simulink model "DT_vehicle_model"  (R2018a)
settings: Solver=FixedStepDiscrete  StartTime=0.0  StopTime=inf  FixedStep=Tsmall  RelTol=1e-3
PreLoadFcn:
  | DT_data
PostLoadFcn:
  | , if any(exist('dsrtsu_mdlpostloadfcn', 'file') == [2, 3, 6]), try dsrtsu_mdlpostloadfcn('Execute', bdroot); catch fprintf('Error in PostLoadFcn (dsrtsu_mdlpostloadfcn) for model "%s":\n %s\n', bdroot, lasterr); end, end,
InitFcn:
  | DT_data
values from neighbouring files (symbols this model uses):
  Bx_ash_f = 11.7    [DT_data.m]
  Bx_ash_r = 11.1    [DT_data.m]
  Bx_snow_f = 10.2    [DT_data.m]
  Bx_snow_r = 9.71    [DT_data.m]
  By_ash_f = 8.86    [DT_data.m]
  By_ash_r = 9.30    (= 9.3)    [DT_data.m]
  By_snow_f = 19.1    [DT_data.m]
  By_snow_r = 20.0    (= 20)    [DT_data.m]
  Cx_ash_f = 1.69    [DT_data.m]
  Cx_ash_r = 1.69    [DT_data.m]
  Cx_snow_f = 1.96    [DT_data.m]
  Cx_snow_r = 1.96    [DT_data.m]
  Cy_ash_f = 1.19    [DT_data.m]
  Cy_ash_r = 1.19    [DT_data.m]
  Cy_snow_f = 0.550    (= 0.55)    [DT_data.m]
  Cy_snow_r = 0.550    (= 0.55)    [DT_data.m]
  D_phi = 16000    [DT_data.m]
  D_theta = 30960    [DT_data.m]
  delta_r = 0    [DT_data.m]
  epsilon = 0.4    [DT_data.m]
  Ex_ash_f = 0.377    [DT_data.m]
  Ex_ash_r = 0.362    [DT_data.m]
  Ex_snow_f = 0.651    [DT_data.m]
  Ex_snow_r = 0.624    [DT_data.m]
  Ey_ash_f = -1.21    [DT_data.m]
  Ey_ash_r = -1.11    [DT_data.m]
  Ey_snow_f = -2.1    [DT_data.m]
  Ey_snow_r = -1.93    [DT_data.m]
  g = 9.81    [DT_data.m]
  h = 0.5    [DT_data.m]
  Iw = 4    [DT_data.m]
  Ixx = 602.1923    [DT_data.m]
  Iyy = 2.7370e+03    (= 2737)    [DT_data.m]
  Izz = 3070    [DT_data.m]
  K_phi = 178000    [DT_data.m]
  K_theta = 363540    [DT_data.m]
  l_f = 1.2110    (= 1.211)    [DT_data.m]
  l_r = 1.4590    (= 1.459)    [DT_data.m]
  m = 1830    [DT_data.m]
  mu_x_ash_f = 1.20    (= 1.2)    [DT_data.m]
  mu_x_ash_r = 1.20    (= 1.2)    [DT_data.m]
  mu_x_snow_f = 0.407    [DT_data.m]
  mu_x_snow_r = 0.409    [DT_data.m]
  mu_y_ash_f = 0.935    [DT_data.m]
  mu_y_ash_r = 0.961    [DT_data.m]
  mu_y_snow_f = 0.383    [DT_data.m]
  mu_y_snow_r = 0.394    [DT_data.m]
  omega0 = 29.1545    [DT_data.m]
  road = 1    [DT_data.m]
  Rw = 0.3430    (= 0.343)    [DT_data.m]
  Ts = 0.001    [DT_data.m]
  Tsmall = 0.001    [DT_data.m]
  Vx0 = 10    [DT_data.m]
  w = 0.7700    (= 0.77)    [DT_data.m]
libraries: simulink x1
(part 1 of 2)
PreSaveFcn:
  | , if any(exist('dsmpb_private', 'file') == [2, 3, 6]), try, dsmpb_private('dsmpb_mdlclblib', 'PreSave', bdroot); catch, disp(lasterr); end, end,
CloseFcn:
  | , if any(exist('dsmpb_private', 'file') == [2, 3, 6]), try, dsmpb_private('dsmpb_mdlclblib', 'Close', bdroot); catch, disp(lasterr); end, end,
Description:
  | Standard RTI1401 template.
  | Supported MATLAB version:  R2017b.
settings Model: Tag=RTI1401  DSRTSU_INTERNAL_RTI_VER=520  DSRTSU_INTERNAL_RTI_TYPE=rti1006  RTICANMMDATA=struct('GeneralSetupData',struct('modelroot','C:\Users\srivats\Documents\MATLAB\DT_vehicle_model','generalsettings',struct('filesettings',struct('destfolder',struct('Name','RTICANMM_FILES','Check',1),'buildfolder',struct('Name','.','Check',1),'AbsDestfolder',struct('Name','C:\Users\srivats\Documents\MATLAB\DT_vehicle_model\RTICANMM_FILES'),'AbsBuildfolder',struct('Name','C:\Users\srivats\Documents\MATLAB\DT_vehicle_model'))),'options',struct('addpaths',1,'rmpaths',1,'addtrcexclusion',logical(1),'cannavigator',struct('checkmonitoring',0),'show_usrtrc',0,'use_usrtrc',0),'advanced',struct('options',[1 1 1 1 1 1 1 1 1 1 1 1 1 1 1 1 1 1 1 1 1 1 1 1 1 1 1 1 1 1 1 1 1 1 1 1 1 1 1 1 1 1 1 1 1 1 1 1 1 1 1 1 1 1 1 1 1 1 1 1 1 1 1 1 1 1 1 1 1 1 1 1 1 1 1 1 1 1 1 1 1 1 1 1 1 1 1 1 1 1 1 1 1 1 1 1 1 1 1 1]),'MPSetup',{{}},'modelname','DT_vehicle_model','block','DT_vehicle_model'))  DSRTSU_INTERNAL_RTIFLEXRAYCONFIG=110  DSRTSU_INTERNAL_RTIFPGA=110  DSMPB_DATASERVER_ModelPortLibVersion1=8  DSMPB_DATASERVER_DataServerVersion1=6  DSMPB_DATASERVER_DataServerStreamVersion1=3  Creator=merl  LastModifiedBy=srivats
settings OptimizationCC: BlockReduction=off  BooleanDataType=off  ConditionallyExecuteInputs=off  OptimizeBlockIOStorage=off  BufferReuse=off  GlobalBufferReuse=off  ExpressionFolding=off  LocalBlockOutputs=off  OptimizeDataStoreBuffers=off  BusAssignmentInplaceUpdate=off
settings DebuggingCC: MultiTaskRateTransMsg=warning  UnknownTsInhSupMsg=error
settings HardwareCC: ProdBitPerPointer=32  ProdBitPerSizeT=32  ProdBitPerPtrDiffT=32  ProdLargestAtomicInteger=Integer  ProdWordSize=32  ProdHWDeviceType=Custom Processor->Custom  TargetIntDivRoundTo=Zero  TargetEndianess=LittleEndian  TargetHWDeviceType=Custom Processor->Custom
settings SFSimCC: MATLABDynamicMemAlloc=off
settings RTWCC: SystemTargetFile=rti1006.tlc  MakeCommand=make_rti  TemplateMakefile=rti1006.tmf  Description=<inactive> dSPACE DS1006 Hardware Platform
settings CodeAppCC: StateflowObjectComments=on
settings STFCustomTargetCC: ParMdlRefBuildCompliant=on  GRTInterface=off  SystemTargetFile=rti1006.tlc
settings GRTTargetCC: TargetLangStandard=C89/C90 (ANSI)  CompOptLevelCompliant=off  ConcurrentExecutionCompliant=off  CombineOutputUpdateFcns=off  MatFileLogging=off  CPPClassGenCompliant=off  UseToolchainInfoCompliant=off
settings ConfigComp: CovMetricSettings=dswe

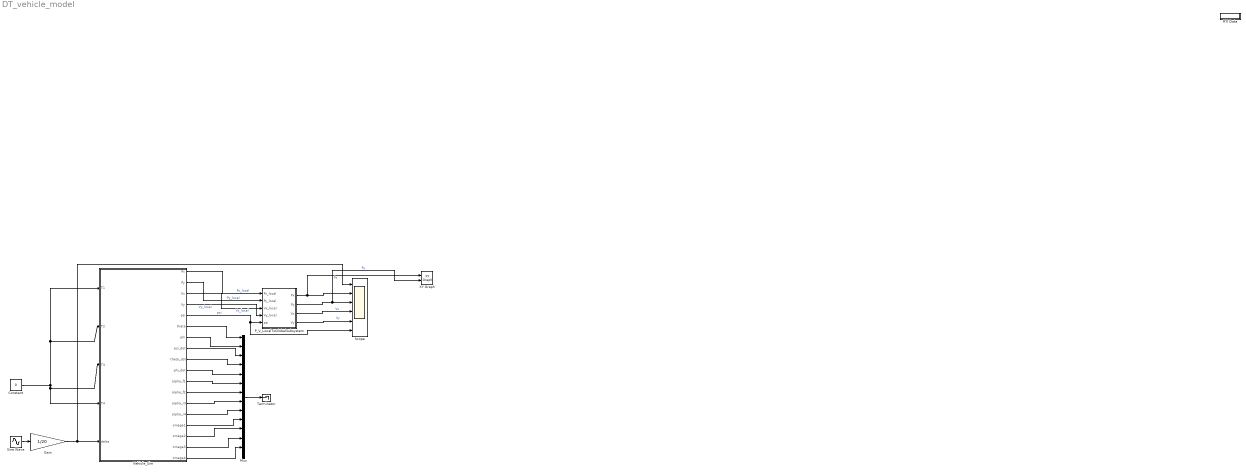
== system DT_vehicle_model ==
  Constant : Constant  Value=0
  Gain : Gain  Gain=1/20
  Mux : Mux  Inputs=14
  P_V_LocalToGlobalSubsystem : Subsystem
  RTI Data : Subsystem  Tag=struct('RTIDataServer',struct('RTIDataServerVs','2','RTIModelDescription','struct(''main'',''DT_vehicle_model'',''sub'','''',''isMp'',0)'))  LoadFcn="if exist('rtidc'), try,  rtidc('DataHostBlockClbLoad', gcbh); catch, disp(['Warning: ''LoadFcn'' for RTI Data block failed: ' lasterr]); end, end,"  mask(RTI_DATA_HOST){}
      mask help:
      | RTI Data Block.
      | This block is used by RTI to store internal model-dependent data.
      | Please keep this block on the root level of the model. Deleting this block will result in data loss.
      |
      | NEVER DELETE OR COPY THIS BLOCK!
      settings: CopyFcn="if exist('rtidc'), try,  rtidc('DataHostBlockClbCopy', gcbh); catch, disp(['Warning: ''CopyFcn'' for RTI Data block failed: ' lasterr]); end, end,"  DeleteFcn="if exist('rtidc'), try,  rtidc('DataHostBlockClbDelete', gcbh); catch, disp(['Warning: ''DeleteFcn'' for RTI Data block failed: ' lasterr]); end, end,"  ModelCloseFcn="if exist('rtidc'), try,  rtidc('DataHostBlockClbModelClose', gcbh); catch, disp(['Warning: ''ModelCloseFcn'' for RTI Data block failed: ' lasterr]); end, end,"  PreSaveFcn="if exist('rtidc'), try,  rtidc('DataHostBlockClbPreSave', gcbh); catch, disp(['Warning: ''PreSaveFcn'' for RTI Data block failed: ' lasterr]); end, end,"  PostSaveFcn="if exist('rtidc'), try,  rtidc('DataHostBlockClbPostSave', gcbh); catch, disp(['Warning: ''PostSaveFcn'' for RTI Data block failed: ' lasterr]); end, end,"  NameChangeFcn="if exist('rtidc'), try,  rtidc('DataHostBlockClbNameChange', gcbh); catch, disp(['Warning: ''NameChangeFcn'' for RTI Data block failed: ' lasterr]); end, end,"
      mask Help:
      | RTI Data Block.
      | This block is used by RTI to store internal model-dependent data.
      | Please keep this block on the root level of the model. Deleting this block will result in data loss.
      | 
      | NEVER DELETE OR COPY THIS BLOCK!
      mask Display:
      | text(0.5, 0.5, 'RTI Data', 'HorizontalAlignment', 'center');
      | plot([1 0]);
  Scope : Scope  NumInputPorts=6
  Sine Wave : Sin  Amplitude=0.5  SampleTime=0
  Terminator : Terminator
  Vehicle_Sim : Subsystem
  XY Graph : simulink/Sinks/XY Graph  xmin=-1000  xmax=1000  ymin=-1000  ymax=1000  st=-1
  wires:
  Vehicle_Sim/6(theta) -> Mux/1
  Vehicle_Sim/7(phi) -> Mux/2
  Vehicle_Sim/8(psi_dot) -> Mux/3
  Vehicle_Sim/9(theta_dot) -> Mux/4
  Vehicle_Sim/10(phi_dot) -> Mux/5
  Vehicle_Sim/11(alpha_f1) -> Mux/6
  Vehicle_Sim/12(alpha_f2) -> Mux/7
  Vehicle_Sim/13(alpha_r3) -> Mux/8
  Vehicle_Sim/14(alpha_r4) -> Mux/9
  Vehicle_Sim/15(omega1) -> Mux/10
  Vehicle_Sim/16(omega2) -> Mux/11
  Vehicle_Sim/17(omega3) -> Mux/12
  Vehicle_Sim/18(omega4) -> Mux/13
  Mux/1 -> Terminator/1
  Sine Wave/1 -> Gain/1
  Vehicle_Sim/1(Px) -> P_V_LocalToGlobalSubsystem/1(Px_local)  "Px_local"
  Vehicle_Sim/2(Py) -> P_V_LocalToGlobalSubsystem/2(Py_local)  "Py_local"
  Vehicle_Sim/3(Vx) -> P_V_LocalToGlobalSubsystem/3(Vx_local)  "Vx_local"
  Vehicle_Sim/4(Vy) -> P_V_LocalToGlobalSubsystem/4(Vy_local)  "Vy_local"
  Vehicle_Sim/5(psi) -> Scope/6, P_V_LocalToGlobalSubsystem/5(psi)  "psi"
  P_V_LocalToGlobalSubsystem/1(Px) -> XY Graph/1, Scope/2  "Px"
  P_V_LocalToGlobalSubsystem/2(Py) -> XY Graph/2, Scope/3  "Py"
  P_V_LocalToGlobalSubsystem/3(Vx) -> Scope/4  "Vx"
  P_V_LocalToGlobalSubsystem/4(Vy) -> Scope/5  "Vy"
  Constant/1 -> Vehicle_Sim/2(T2), Vehicle_Sim/1(T1), Vehicle_Sim/4(T4), Vehicle_Sim/3(T3)
  Gain/1 -> Scope/1, Vehicle_Sim/5("delta ")

== system DT_vehicle_model/P_V_LocalToGlobalSubsystem ==
  Px_local : Inport  OutDataTypeStr=double  SampleTime=Ts
  Py_local : Inport  Port=2  OutDataTypeStr=double  SampleTime=Ts
  Vx_local : Inport  Port=3  OutDataTypeStr=double  SampleTime=Ts
  Vy_local : Inport  Port=4  OutDataTypeStr=double  SampleTime=Ts
  psi : Inport  Port=5  OutDataTypeStr=double  SampleTime=Ts
  Add : Sum  Inputs=+-
  Add1 : Sum
  Add2 : Sum  Inputs=+-
  Add3 : Sum
  Cos : Trigonometry  Operator=cos
  Product{,1..7} (8 alike) : Product
  Sin : Trigonometry
  Px : Outport  OutDataTypeStr=double  SampleTime=Ts
  Py : Outport  Port=2  OutDataTypeStr=double  SampleTime=Ts
  Vx : Outport  Port=3  OutDataTypeStr=double  SampleTime=Ts
  Vy : Outport  Port=4  OutDataTypeStr=double  SampleTime=Ts
  wires:
  Px_local/1 -> Product6/1, Product4/1  "Px_local"
  Py_local/1 -> Product7/1, Product5/1  "Py_local"
  Vx_local/1 -> Product2/1, Product/2  "Vx_local"
  Product5/1 -> Add2/2
  Product4/1 -> Add2/1
  Add2/1 -> Px/1  "Px"
  Product7/1 -> Add3/2
  Vy_local/1 -> Product3/1, Product1/2  "Vy_local"
  psi/1 -> Sin/1, Cos/1  "psi"
  Cos/1 -> Product3/2, Product/1, Product7/2, Product4/2  "cosPsi"
  Add3/1 -> Py/1  "Py"
  Product2/1 -> Add1/1
  Product1/1 -> Add/2
  Add/1 -> Vx/1  "Vx"
  Add1/1 -> Vy/1  "Vy"
  Product6/1 -> Add3/1
  Product3/1 -> Add1/2
  Product/1 -> Add/1
  Sin/1 -> Product2/2, Product1/1, Product6/2, Product5/2  "sinPsi"

== system DT_vehicle_model/RTI Data ==
  RTI Data Store : Subsystem  Tag="struct('private',struct('version',struct('dsVer',uint32(2),'dsVerCreation',uint32(2),'RTI',struct('ver','7.10','type','RTI1006')),'access',struct('type','Model','isPerm',1,'created',['01-Nov-2018 15:30:42'],'modified',['05-Apr-2019 15:16:55'],'location','')),'public',struct('main',struct('data',[]),'sub',struct('name',{{'DT_vehicle_model'}},'data',{{struct('TH',struct('thTaskInfo',struct('taskType',{'TIMER','HWINT','TMRINT','SWINT','GLINT'},'tasksNumOf',{1,0,0,0,0},'srcIds',{{'TIMERA'},{},{},{},{}},'taskNames',{{['Timer Task 1']},{},{},{},{}})),'th_tc',struct('dataType','TASK','taskGroupId','','taskGroupList',{{}},'taskSchedulingPolicy','FCFS','taskType','TIMER','blkh',-1,'srcId','TIMERA','srcSgnName',['Timer A interrupt'],'srcCpuName','','taskName',['Timer Task 1  [0.001] s'],'taskNameDisplayExt','','smplTime',0.001,'smplTimeOffs',0,'hasFixedPriority',0,'priority',1,'hasFixedOvc',0,'ovcType',1,'ovcMax',1),'tc_th',struct('dataType','TASK','taskGroupId','','taskGroupList',{{}},'taskSchedulingPolicy','FCFS','taskType','TIMER','blkh',-1,'srcId','TIMERA','srcSgnName',['Timer A interrupt'],'srcCpuName','','taskName',['Timer Task 1  [0.001] s'],'taskNameDisplayExt','','smplTime',0.001,'smplTimeOffs',0,'hasFixedPriority',0,'priority',1,'hasFixedOvc',0,'ovcType',1,'ovcMax',1))}})))"  mask(RTI_DATA_STORE){}
      mask help:
      | RTI Data Store Block. This block is used by RTI to store internal model dependent data. Deleting this block will result in data loss.
      |
      | NEVER DELETE, COPY, OR MODIFY THIS BLOCK!
      mask Help:
      | RTI Data Store Block. This block is used by RTI to store internal model dependent data. Deleting this block will result in data loss.
      | 
      | NEVER DELETE, COPY, OR MODIFY THIS BLOCK!
      mask Display: text(0.5, 0.5, ' ', 'HorizontalAlignment', 'center');

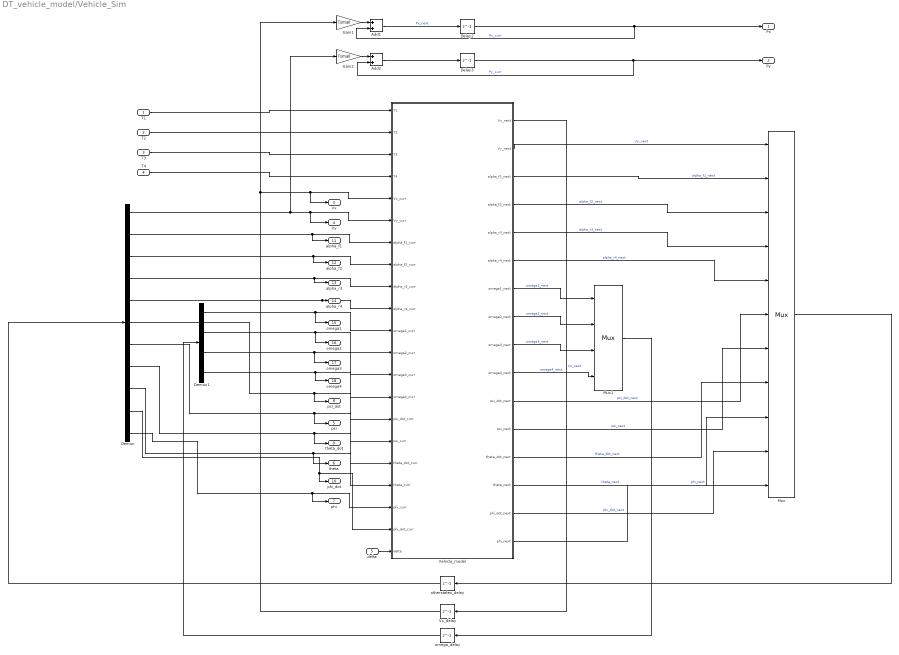
== system DT_vehicle_model/Vehicle_Sim ==
  T1 : Inport  OutDataTypeStr=double  SampleTime=Ts
  T2 : Inport  Port=2  OutDataTypeStr=double  SampleTime=Ts
  T3 : Inport  Port=3  OutDataTypeStr=double  SampleTime=Ts
  T4 : Inport  Port=4  OutDataTypeStr=double  SampleTime=Ts
  "delta " : Inport  Port=5
  Add1 : Sum
  Add2 : Sum
  Delay2 : Delay  DelayLength=1  SampleTime=Tsmall
  Delay3 : Delay  DelayLength=1  SampleTime=Tsmall
  Demux : Demux  Outputs=11
  Demux1 : Demux
  Gain1 : Gain  Gain=Tsmall
  Gain2 : Gain  Gain=Tsmall
  Mux : Mux  Inputs=11
      settings: DisplayOption=signals
  Mux1 : Mux
      settings: DisplayOption=signals
  Vehicle_model : Subsystem
  Vx_delay : Delay  DelayLength=1  InitialCondition=Vx0  SampleTime=Tsmall
  omega_delay : Delay  DelayLength=1  InitialCondition=omega0*ones(4,1)  SampleTime=Tsmall
  otherstates_delay : Delay  DelayLength=1  InitialCondition=zeros(11,1)  SampleTime=Tsmall
  Px : Outport  OutDataTypeStr=double  SampleTime=Tsmall
  Py : Outport  Port=2  OutDataTypeStr=double  SampleTime=Tsmall
  Vx : Outport  Port=3  OutDataTypeStr=double  SampleTime=Tsmall
  Vy : Outport  Port=4  OutDataTypeStr=double  SampleTime=Tsmall
  psi : Outport  Port=5  OutDataTypeStr=double  SampleTime=Tsmall
  theta : Outport  Port=6  OutDataTypeStr=double  SampleTime=Tsmall
  phi : Outport  Port=7  OutDataTypeStr=double  SampleTime=Tsmall
  psi_dot : Outport  Port=8  OutDataTypeStr=double  SampleTime=Tsmall
  theta_dot : Outport  Port=9  OutDataTypeStr=double  SampleTime=Tsmall
  phi_dot : Outport  Port=10  OutDataTypeStr=double  SampleTime=Tsmall
  alpha_f1 : Outport  Port=11  OutDataTypeStr=double  SampleTime=Tsmall
  alpha_f2 : Outport  Port=12  OutDataTypeStr=double  SampleTime=Tsmall
  alpha_r3 : Outport  Port=13  OutDataTypeStr=double  SampleTime=Tsmall
  alpha_r4 : Outport  Port=14  OutDataTypeStr=double  SampleTime=Tsmall
  omega1 : Outport  Port=15  OutDataTypeStr=double  SampleTime=Tsmall
  omega2 : Outport  Port=16  OutDataTypeStr=double  SampleTime=Tsmall
  omega3 : Outport  Port=17  OutDataTypeStr=double  SampleTime=Tsmall
  omega4 : Outport  Port=18  OutDataTypeStr=double  SampleTime=Tsmall
  wires:
  Vehicle_model/14(theta_next) -> Mux/9  "theta_next"
  Vehicle_model/12(psi_next) -> Mux/7  "psi_next"
  Vehicle_model/11(psi_dot_next) -> Mux/6  "psi_dot_next"
  Vehicle_model/15(phi_dot_next) -> Mux/10  "phi_dot_next"
  Mux/1 -> otherstates_delay/1
  Vehicle_model/3(alpha_f1_next) -> Mux/2  "alpha_f1_next"
  Vehicle_model/5(alpha_r3_next) -> Mux/4  "alpha_r3_next"
  Vehicle_model/9(omega3_next) -> Mux1/3  "omega3_next"
  Vehicle_model/8(omega2_next) -> Mux1/2  "omega2_next"
  Vehicle_model/13(theta_dot_next) -> Mux/8  "theta_dot_next"
  Vehicle_model/4(alpha_f2_next) -> Mux/3  "alpha_f2_next"
  Vehicle_model/6(alpha_r4_next) -> Mux/5  "alpha_r4_next"
  Vehicle_model/10(omega4_next) -> Mux1/4  "omega4_next"
  Vehicle_model/1(Vx_next) -> Vx_delay/1  "Vx_next"
  Demux/1 -> Gain2/1, Vy/1, Vehicle_model/6(Vy_curr)
  Vehicle_model/7(omega1_next) -> Mux1/1  "omega1_next"
  Demux1/3 -> omega3/1, Vehicle_model/13(omega3_curr)
  Demux/5 -> Vehicle_model/10(alpha_r4_curr), alpha_r4/1
  Demux/8 -> theta_dot/1, Vehicle_model/17(theta_dot_curr)
  Vehicle_model/16(phi_next) -> Mux/11  "phi_next"
  Vehicle_model/2(Vy_next) -> Mux/1  "Vy_next"
  T1/1 -> Vehicle_model/1(T1)
  Add2/1 -> Delay3/1
  Delay3/1 -> Py/1, Add2/2  "Py_curr"
  Add1/1 -> Delay2/1  "Px_next"
  Delay2/1 -> Px/1, Add1/2  "Px_curr"
  Gain1/1 -> Add1/1
  Gain2/1 -> Add2/1
  T3/1 -> Vehicle_model/3(T3)
  T4/1 -> Vehicle_model/4(T4)
  T2/1 -> Vehicle_model/2(T2)
  otherstates_delay/1 -> Demux/1
  Demux/4 -> Vehicle_model/9(alpha_r3_curr), alpha_r3/1
  Demux/11 -> phi/1, Vehicle_model/19(phi_curr)
  Demux/2 -> Vehicle_model/7(alpha_f1_curr), alpha_f1/1
  Demux/3 -> Vehicle_model/8(alpha_f2_curr), alpha_f2/1
  Demux1/4 -> omega4/1, Vehicle_model/14(omega4_curr)
  Demux/7 -> psi/1, Vehicle_model/16(psi_curr)
  Demux/9 -> theta/1, Vehicle_model/18(theta_curr)
  Demux/10 -> phi_dot/1, Vehicle_model/20(phi_dot_curr)
  Demux/6 -> psi_dot/1, Vehicle_model/15(psi_dot_curr)
  Demux1/2 -> omega2/1, Vehicle_model/12(omega2_curr)
  Vx_delay/1 -> Vx/1, Vehicle_model/5(Vx_curr), Gain1/1
  Demux1/1 -> omega1/1, Vehicle_model/11(omega1_curr)
  Mux1/1 -> omega_delay/1
  omega_delay/1 -> Demux1/1
  "delta "/1 -> Vehicle_model/21(delta)

== system DT_vehicle_model/RTI Data/RTI Data Store ==
  RTI Data Store : Subsystem  mask(RTI_DATA_STORE){}
      mask help:
      | RTI Data Store Block. This block is used by RTI to store internal model dependent data. Deleting this block will result in data loss.
      |
      | NEVER DELETE, COPY, OR MODIFY THIS BLOCK!
      mask Help:
      | RTI Data Store Block. This block is used by RTI to store internal model dependent data. Deleting this block will result in data loss.
      | 
      | NEVER DELETE, COPY, OR MODIFY THIS BLOCK!
      mask Display: text(0.5, 0.5, ' ', 'HorizontalAlignment', 'center');

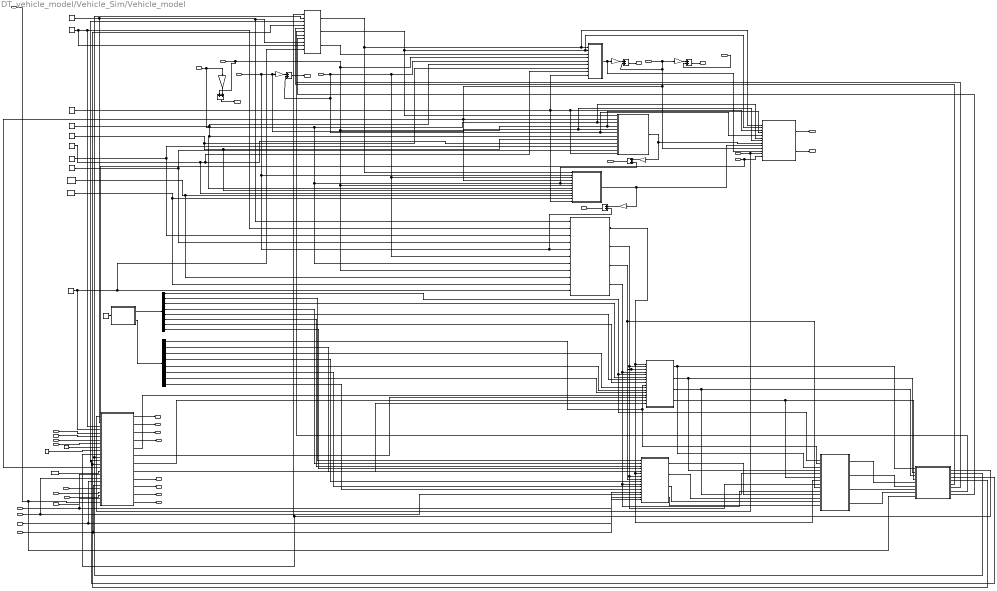
== system DT_vehicle_model/Vehicle_Sim/Vehicle_model ==
  T1 : Inport  OutDataTypeStr=double  SampleTime=Ts
  T2 : Inport  Port=2  OutDataTypeStr=double  SampleTime=Ts
  T3 : Inport  Port=3  OutDataTypeStr=double  SampleTime=Ts
  T4 : Inport  Port=4  OutDataTypeStr=double  SampleTime=Ts
  Vx_curr : Inport  Port=5  OutDataTypeStr=double  SampleTime=Tsmall
  Vy_curr : Inport  Port=6  OutDataTypeStr=double  SampleTime=Tsmall
  alpha_f1_curr : Inport  Port=7  OutDataTypeStr=double  SampleTime=Tsmall
  alpha_f2_curr : Inport  Port=8  OutDataTypeStr=double  SampleTime=Tsmall
  alpha_r3_curr : Inport  Port=9  OutDataTypeStr=double  SampleTime=Tsmall
  alpha_r4_curr : Inport  Port=10  OutDataTypeStr=double  SampleTime=Tsmall
  omega1_curr : Inport  Port=11  OutDataTypeStr=double  SampleTime=Tsmall
  omega2_curr : Inport  Port=12  OutDataTypeStr=double  SampleTime=Tsmall
  omega3_curr : Inport  Port=13  OutDataTypeStr=double  SampleTime=Tsmall
  omega4_curr : Inport  Port=14  OutDataTypeStr=double  SampleTime=Tsmall
  psi_dot_curr : Inport  Port=15  OutDataTypeStr=double  SampleTime=Tsmall
  psi_curr : Inport  Port=16  OutDataTypeStr=double  SampleTime=Tsmall
  theta_dot_curr : Inport  Port=17  OutDataTypeStr=double  SampleTime=Tsmall
  theta_curr : Inport  Port=18  OutDataTypeStr=double  SampleTime=Tsmall
  phi_curr : Inport  Port=19  OutDataTypeStr=double  SampleTime=Tsmall
  phi_dot_curr : Inport  Port=20  OutDataTypeStr=double  SampleTime=Tsmall
  delta : Inport  Port=21  OutDataTypeStr=double  SampleTime=Tsmall
  Add{,1..5} (6 alike) : Sum
  D_phi : Constant  Value=D_phi
  D_theta : Constant  Value=D_theta
  Demux1 : Demux  Outputs=8
  Demux2 : Demux  Outputs=8
  F_M_subsystem : Subsystem
  Fx0_Subsystem : Subsystem
  Fy0_Subsystem : Subsystem
  Fy0_to_Fy_subsystem : Subsystem
  Fz_Subsystem : Subsystem
  Gain{,1..5} (6 alike) : Gain  Gain=Tsmall
  Iw : Constant  Value=Iw
  Ixx : Constant  Value=Ixx
  Iyy : Constant  Value=Iyy
  Izz : Constant  Value=Izz
  K_phi : Constant  Value=K_phi
  K_theta : Constant  Value=K_theta
  Pacjeka_parameters_Subsystem : Subsystem
  Rw : Constant  Value=Rw
  Vx_Vy_Subsystem : Subsystem
  epsilon : Constant  Value=epsilon
  h : Constant  Value=h
  l_f : Constant  Value=l_f
  l_r : Constant  Value=l_r
  local_to_global_Fx_Fy_Subsystem : Subsystem
  omega_alpha_and_k_values_subsystem : Subsystem
  phi_subsystem : Subsystem
  psi_subsystem : Subsystem
  surface : Constant  Value=road
  theta_subsystem : Subsystem
  w : Constant  Value=w
  Vx_next : Outport  OutDataTypeStr=double  SampleTime=Tsmall
  Vy_next : Outport  Port=2  OutDataTypeStr=double  SampleTime=Tsmall
  alpha_f1_next : Outport  Port=3  OutDataTypeStr=double  SampleTime=Tsmall
  alpha_f2_next : Outport  Port=4  OutDataTypeStr=double  SampleTime=Tsmall
  alpha_r3_next : Outport  Port=5  OutDataTypeStr=double  SampleTime=Tsmall
  alpha_r4_next : Outport  Port=6  OutDataTypeStr=double  SampleTime=Tsmall
  omega1_next : Outport  Port=7  OutDataTypeStr=double  SampleTime=Tsmall
  omega2_next : Outport  Port=8  OutDataTypeStr=double  SampleTime=Tsmall
  omega3_next : Outport  Port=9  OutDataTypeStr=double  SampleTime=Tsmall
  omega4_next : Outport  Port=10  OutDataTypeStr=double  SampleTime=Tsmall
  psi_dot_next : Outport  Port=11  OutDataTypeStr=double  SampleTime=Tsmall
  psi_next : Outport  Port=12  OutDataTypeStr=double  SampleTime=Tsmall
  theta_dot_next : Outport  Port=13  OutDataTypeStr=double  SampleTime=Tsmall
  theta_next : Outport  Port=14  OutDataTypeStr=double  SampleTime=Tsmall
  phi_dot_next : Outport  Port=15  OutDataTypeStr=double  SampleTime=Tsmall
  phi_next : Outport  Port=16  OutDataTypeStr=double  SampleTime=Tsmall
  wires:
  Add/1 -> psi_dot_next/1
  Gain4/1 -> Add4/1
  Gain5/1 -> Add5/2
  Add4/1 -> phi_dot_next/1
  Add5/1 -> phi_next/1
  omega1_curr/1 -> omega_alpha_and_k_values_subsystem/22(omega1_curr)
  omega3_curr/1 -> omega_alpha_and_k_values_subsystem/24(omega3_curr)
  omega_alpha_and_k_values_subsystem/11(omega3_next) -> omega3_next/1
  omega_alpha_and_k_values_subsystem/12(omega4_next) -> omega4_next/1
  F_M_subsystem/2(FY) -> phi_subsystem/1(FY), Vx_Vy_Subsystem/2(FY), psi_subsystem/2(FY)  "Fy"
  theta_curr/1 -> Add3/2, Vx_Vy_Subsystem/5(theta), phi_subsystem/6(theta), psi_subsystem/5(theta), Fz_Subsystem/6(theta), theta_subsystem/3(theta)
  Ixx/1 -> psi_subsystem/6(Ixx), theta_subsystem/7(Ixx), phi_subsystem/7(Ixx)  "Ixx"
  phi_dot_curr/1 -> Vx_Vy_Subsystem/6(phi_dot), phi_subsystem/3(phi_dot), Add4/2, theta_subsystem/5(phi_dot), Fz_Subsystem/7(phi_dot), Gain5/1  "phi_dot"
  Izz/1 -> theta_subsystem/9(Izz), psi_subsystem/8(Izz), phi_subsystem/9(Izz)  "Izz"
  theta_subsystem/1(theta_ddot) -> Vx_Vy_Subsystem/9(theta_ddot), Gain2/1  "theta_ddot"
  K_phi/1 -> Fz_Subsystem/3(k_phi), phi_subsystem/10(K_phi)  "k_phi"
  F_M_subsystem/1(FX) -> theta_subsystem/1(FX), Vx_Vy_Subsystem/1(FX), psi_subsystem/1(FX)  "Fx"
  phi_curr/1 -> Add5/1, Fz_Subsystem/8(phi), theta_subsystem/6(phi), Vx_Vy_Subsystem/4(phi), phi_subsystem/4(phi), psi_subsystem/4(phi)
  theta_dot_curr/1 -> Gain3/1, Vx_Vy_Subsystem/7(theta_dot), phi_subsystem/5(theta_dot), theta_subsystem/2(theta_dot), Add2/2, Fz_Subsystem/5(theta_dot)
  F_M_subsystem/3(Mz) -> psi_subsystem/3(MZ)  "MZ"
  psi_subsystem/1(psi_ddot) -> Gain/1, Vx_Vy_Subsystem/11(psi_ddot)  "psi_ddot"
  phi_subsystem/1(phi_ddot) -> Vx_Vy_Subsystem/8(phi_ddot), Gain4/1  "phi_ddot"
  Iyy/1 -> psi_subsystem/7(Iyy), theta_subsystem/8(Iyy), phi_subsystem/8(Iyy)  "Iyy"
  D_theta/1 -> Fz_Subsystem/10(D_theta), theta_subsystem/11(D_theta)  "D_theta"
  Pacjeka_parameters_Subsystem/1(front) -> Demux1/1
  w/1 -> omega_alpha_and_k_values_subsystem/5(w), F_M_subsystem/11(w), Fz_Subsystem/11(w)  "w"
  Demux1/4 -> Fy0_Subsystem/2(C_y_f)  "C_y_f"
  Demux1/2 -> Fy0_Subsystem/1(mu_y_f)  "mu_y_f"
  Fz_Subsystem/2(Fz2) -> Fy0_to_Fy_subsystem/8(Fz2), Fy0_Subsystem/7(Fz2), Fx0_Subsystem/2(Fz2)  "Fz2"
  Demux2/1 -> Fy0_to_Fy_subsystem/2(mu_x_r), Fx0_Subsystem/9(mu_x_r)  "mu_x_r"
  omega_alpha_and_k_values_subsystem/6(k_f2) -> Fx0_Subsystem/14(k_f2)  "k_f2"
  Demux1/8 -> Fy0_Subsystem/4(E_y_f)  "E_y_f"
  Demux1/6 -> Fy0_Subsystem/3(B_y_f)  "B_y_f"
  surface/1 -> Pacjeka_parameters_Subsystem/1(surface_condition)
  l_r/1 -> F_M_subsystem/10(l_r), omega_alpha_and_k_values_subsystem/4(l_r), Fz_Subsystem/2(l_r)  "l_r"
  Fz_Subsystem/4(Fz4) -> Fy0_to_Fy_subsystem/10(Fz4), Fy0_Subsystem/10(Fz4), Fx0_Subsystem/4(Fz4)  "Fz4"
  Demux1/5 -> Fx0_Subsystem/7(B_x_f)  "B_x_f"
  Demux1/7 -> Fx0_Subsystem/8(E_x_f)  "E_x_f"
  D_phi/1 -> Fz_Subsystem/4(d_phi), phi_subsystem/11(D_phi)  "d_phi"
  omega_alpha_and_k_values_subsystem/5(k_f1) -> Fx0_Subsystem/13(k_f1)  "k_f1"
  Demux1/1 -> Fy0_to_Fy_subsystem/1(mu_x_f), Fx0_Subsystem/5(mu_x_f)  "mu_x_f"
  omega_alpha_and_k_values_subsystem/7(k_r3) -> Fx0_Subsystem/15(k_r3)  "k_r3"
  l_f/1 -> omega_alpha_and_k_values_subsystem/3(l_f), F_M_subsystem/9(l_f), Fz_Subsystem/1(l_f)  "l_f"
  K_theta/1 -> Fz_Subsystem/9(K_theta), theta_subsystem/10(K_theta)  "K_theta"
  Demux2/3 -> Fx0_Subsystem/10(C_x_r)  "C_x_r"
  Demux2/7 -> Fx0_Subsystem/12(E_x_r)  "E_x_r"
  Pacjeka_parameters_Subsystem/2(rear) -> Demux2/1
  omega_alpha_and_k_values_subsystem/8(k_r4) -> Fx0_Subsystem/16(k_r4)  "k_r4"
  Fx0_Subsystem/1(Fx01) -> local_to_global_Fx_Fy_Subsystem/1(local_Fx1), Fy0_to_Fy_subsystem/3(Fx01)  "Fx01"
  Demux1/3 -> Fx0_Subsystem/6(C_x_f)  "C_x_f"
  Demux2/5 -> Fx0_Subsystem/11(B_x_r)  "B_x_r"
  Fz_Subsystem/1(Fz1) -> Fx0_Subsystem/1(Fz1), Fy0_to_Fy_subsystem/7(Fz1), Fy0_Subsystem/6(Fz1)  "Fz1"
  Demux2/6 -> Fy0_Subsystem/11(B_y_r)  "B_y_r"
  Fz_Subsystem/3(Fz3) -> Fy0_to_Fy_subsystem/9(Fz3), Fx0_Subsystem/3(Fz3), Fy0_Subsystem/8(Fz3)  "Fz3"
  local_to_global_Fx_Fy_Subsystem/6(Fy2) -> F_M_subsystem/6(Fy2)  "Fy2"
  T4/1 -> omega_alpha_and_k_values_subsystem/9(T4)
  Demux2/8 -> Fy0_Subsystem/12(E_y_r)  "E_y_r"
  Fy0_Subsystem/4(Fy04) -> Fy0_to_Fy_subsystem/14(Fy04)  "Fy04"
  alpha_f1_curr/1 -> omega_alpha_and_k_values_subsystem/18(alpha_f1_curr), Fy0_Subsystem/13(alpha_f1)
  epsilon/1 -> omega_alpha_and_k_values_subsystem/17(epsilon)
  Vx_Vy_Subsystem/1(Vx_next) -> Vx_next/1
  Fx0_Subsystem/4(Fx04) -> local_to_global_Fx_Fy_Subsystem/4(local_Fx4), Fy0_to_Fy_subsystem/6(Fx04)  "Fx04"
  alpha_f2_curr/1 -> Fy0_Subsystem/14(alpha_f2), omega_alpha_and_k_values_subsystem/19(alpha_f2_curr)
  Fy0_Subsystem/1(Fy01) -> Fy0_to_Fy_subsystem/11(Fy01)  "Fy01"
  Fy0_Subsystem/2(Fy02) -> Fy0_to_Fy_subsystem/12(Fy02)  "Fy02"
  Demux2/4 -> Fy0_Subsystem/9(C_y_r)  "C_y_r"
  local_to_global_Fx_Fy_Subsystem/5(Fy1) -> F_M_subsystem/5(Fy1)  "Fy1"
  Fx0_Subsystem/3(Fx03) -> Fy0_to_Fy_subsystem/5(Fx03), local_to_global_Fx_Fy_Subsystem/3(local_Fx3)  "Fx03"
  local_to_global_Fx_Fy_Subsystem/7(Fy3) -> F_M_subsystem/7(Fy3)  "Fy3"
  Rw/1 -> omega_alpha_and_k_values_subsystem/10(Rw)
  h/1 -> Vx_Vy_Subsystem/3(h), phi_subsystem/12(h), psi_subsystem/9(h), theta_subsystem/12(h)  "h"
  Fx0_Subsystem/2(Fx02) -> local_to_global_Fx_Fy_Subsystem/2(local_Fx2), Fy0_to_Fy_subsystem/4(Fx02)
  local_to_global_Fx_Fy_Subsystem/8(Fy4) -> F_M_subsystem/8(Fy4)  "Fy4"
  T3/1 -> omega_alpha_and_k_values_subsystem/8(T3)
  T1/1 -> omega_alpha_and_k_values_subsystem/6(T1)
  Iw/1 -> omega_alpha_and_k_values_subsystem/11(Iw)
  T2/1 -> omega_alpha_and_k_values_subsystem/7(T2)
  alpha_r4_curr/1 -> Fy0_Subsystem/16(alpha_r4), omega_alpha_and_k_values_subsystem/21(alpha_r4_curr)
  Fy0_Subsystem/3(Fy03) -> Fy0_to_Fy_subsystem/13(Fy03)  "Fy03"
  Demux2/2 -> Fy0_Subsystem/5(mu_y_r)  "mu_y_r"
  alpha_r3_curr/1 -> Fy0_Subsystem/15(alpha_r3), omega_alpha_and_k_values_subsystem/20(alpha_r3_curr)
  Vy_curr/1 -> omega_alpha_and_k_values_subsystem/2(Vy), Vx_Vy_Subsystem/13(Vy_curr)
  omega_alpha_and_k_values_subsystem/3(alpha_r3_next) -> alpha_r3_next/1
  Vx_curr/1 -> omega_alpha_and_k_values_subsystem/1(Vx), Vx_Vy_Subsystem/12(Vx_curr)
  omega_alpha_and_k_values_subsystem/1(alpha_f1_next) -> alpha_f1_next/1  "alpha_f1"
  omega_alpha_and_k_values_subsystem/4(alpha_r4_next) -> alpha_r4_next/1  "alpha_r4"
  Vx_Vy_Subsystem/2(Vy_next) -> Vy_next/1
  omega_alpha_and_k_values_subsystem/2(alpha_f2_next) -> alpha_f2_next/1  "alpha_f2"
  psi_dot_curr/1 -> Gain1/1, Add/2, Vx_Vy_Subsystem/10(psi_dot), omega_alpha_and_k_values_subsystem/16(psi_dot), theta_subsystem/4(psi_dot), phi_subsystem/2(psi_dot)  "psi_dot"
  Gain1/1 -> Add1/1
  psi_curr/1 -> Add1/2
  omega4_curr/1 -> omega_alpha_and_k_values_subsystem/25(omega4_curr)
  omega_alpha_and_k_values_subsystem/10(omega2_next) -> omega2_next/1
  omega2_curr/1 -> omega_alpha_and_k_values_subsystem/23(omega2_curr)
  Gain3/1 -> Add3/1
  Gain2/1 -> Add2/1
  Gain/1 -> Add/1
  Add3/1 -> theta_next/1
  Add2/1 -> theta_dot_next/1
  Add1/1 -> psi_next/1
  omega_alpha_and_k_values_subsystem/9(omega1_next) -> omega1_next/1
  delta/1 -> local_to_global_Fx_Fy_Subsystem/9(delta_f2), omega_alpha_and_k_values_subsystem/26(delta_f2)  "delta_f2"
  Fy0_to_Fy_subsystem/1(local_Fy1) -> local_to_global_Fx_Fy_Subsystem/5(local_Fy1)  "Fy1"
  Fy0_to_Fy_subsystem/2(local_Fy2) -> local_to_global_Fx_Fy_Subsystem/6(local_Fy2)  "Fy2"
  Fy0_to_Fy_subsystem/3(local_Fy3) -> local_to_global_Fx_Fy_Subsystem/7(local_Fy3)  "Fy3"
  Fy0_to_Fy_subsystem/4(lcoal_Fy4) -> local_to_global_Fx_Fy_Subsystem/8(local_Fy4)  "Fy4"
  local_to_global_Fx_Fy_Subsystem/1(Fx1) -> omega_alpha_and_k_values_subsystem/12(Fx1), F_M_subsystem/1(Fx1)  "Fx1"
  local_to_global_Fx_Fy_Subsystem/2(Fx2) -> omega_alpha_and_k_values_subsystem/13(Fx2), F_M_subsystem/2(Fx2)  "Fx2"
  local_to_global_Fx_Fy_Subsystem/3(Fx3) -> F_M_subsystem/3(Fx3), omega_alpha_and_k_values_subsystem/14(Fx3)  "Fx3"
  local_to_global_Fx_Fy_Subsystem/4(Fx4) -> F_M_subsystem/4(Fx4), omega_alpha_and_k_values_subsystem/15(Fx4)  "Fx4"

== system DT_vehicle_model/RTI Data/RTI Data Store/RTI Data Store ==
  RTI Data Store : Subsystem  mask(RTI_DATA_STORE){}
      mask help:
      | RTI Data Store Block. This block is used by RTI to store internal model dependent data. Deleting this block will result in data loss.
      |
      | NEVER DELETE, COPY, OR MODIFY THIS BLOCK!
      mask Help:
      | RTI Data Store Block. This block is used by RTI to store internal model dependent data. Deleting this block will result in data loss.
      | 
      | NEVER DELETE, COPY, OR MODIFY THIS BLOCK!
      mask Display: text(0.5, 0.5, ' ', 'HorizontalAlignment', 'center');

== system DT_vehicle_model/Vehicle_Sim/Vehicle_model/F_M_subsystem ==
  Fx1 : Inport  OutDataTypeStr=double  SampleTime=Ts
  Fx2 : Inport  Port=2  OutDataTypeStr=double  SampleTime=Ts
  Fx3 : Inport  Port=3  OutDataTypeStr=double  SampleTime=Ts
  Fx4 : Inport  Port=4  OutDataTypeStr=double  SampleTime=Ts
  Fy1 : Inport  Port=5  OutDataTypeStr=double  SampleTime=Ts
  Fy2 : Inport  Port=6  OutDataTypeStr=double  SampleTime=Ts
  Fy3 : Inport  Port=7  OutDataTypeStr=double  SampleTime=Ts
  Fy4 : Inport  Port=8  OutDataTypeStr=double  SampleTime=Ts
  l_f : Inport  Port=9  OutDataTypeStr=double  SampleTime=Ts
  l_r : Inport  Port=10  OutDataTypeStr=double  SampleTime=Ts
  w : Inport  Port=11  OutDataTypeStr=double  SampleTime=Ts
  Add : Sum  Inputs=++++
  Add1 : Sum  Inputs=++++
  Add2 : Sum  Inputs=++--
  Add3 : Sum
  Add4 : Sum
  Product{,1..3} (4 alike) : Product
  Subtract : Sum  Inputs=+-
  Subtract1 : Sum
  FX : Outport
  FY : Outport  Port=2
  Mz : Outport  Port=3
  wires:
  Fy2/1 -> Add3/2, Add1/2  "Fy2"
  Fx3/1 -> Subtract1/1, Add/1
  Fx4/1 -> Subtract1/2, Add/2
  Fx1/1 -> Subtract/2, Add/3  "Fx1"
  Fx2/1 -> Subtract/1, Add/4  "Fx2"
  Add/1 -> FX/1
  Fy1/1 -> Add3/1, Add1/1  "Fy1"
  Fy3/1 -> Add4/1, Add1/3
  Fy4/1 -> Add4/2, Add1/4
  Add1/1 -> FY/1
  Add2/1 -> Mz/1
  Add3/1 -> Product/1
  l_f/1 -> Product/2
  Product/1 -> Add2/1
  Subtract/1 -> Product1/2
  w/1 -> Product3/2, Product1/1
  Product1/1 -> Add2/2
  Add4/1 -> Product2/1
  l_r/1 -> Product2/2
  Product2/1 -> Add2/3
  Subtract1/1 -> Product3/1
  Product3/1 -> Add2/4

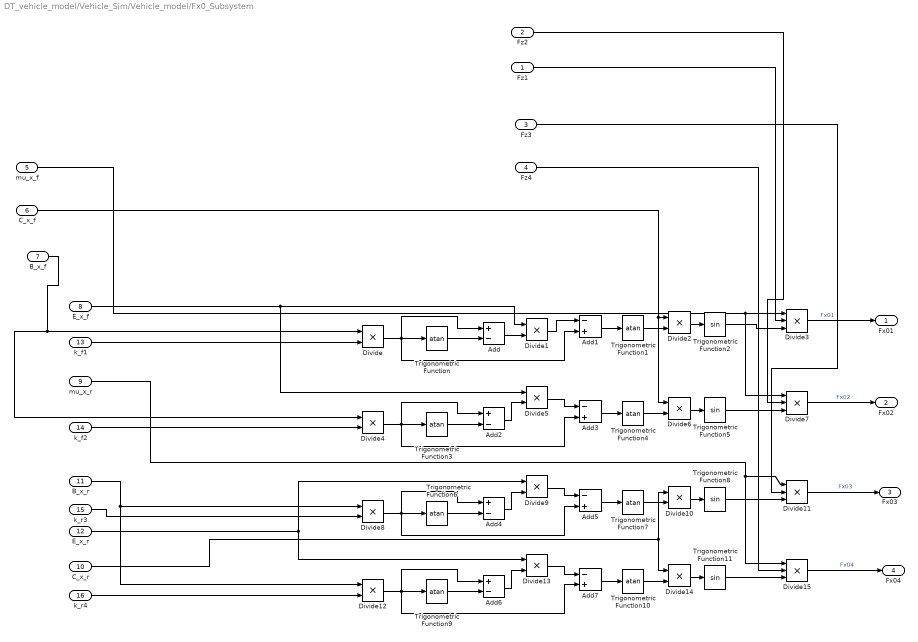
== system DT_vehicle_model/Vehicle_Sim/Vehicle_model/Fx0_Subsystem ==
  Fz1 : Inport  OutDataTypeStr=double  SampleTime=Ts
  Fz2 : Inport  Port=2  OutDataTypeStr=double  SampleTime=Ts
  Fz3 : Inport  Port=3  OutDataTypeStr=double  SampleTime=Ts
  Fz4 : Inport  Port=4  OutDataTypeStr=double  SampleTime=Ts
  mu_x_f : Inport  Port=5
  C_x_f : Inport  Port=6
  B_x_f : Inport  Port=7
  E_x_f : Inport  Port=8
  mu_x_r : Inport  Port=9
  C_x_r : Inport  Port=10
  B_x_r : Inport  Port=11
  E_x_r : Inport  Port=12
  k_f1 : Inport  Port=13
  k_f2 : Inport  Port=14
  k_r3 : Inport  Port=15
  k_r4 : Inport  Port=16
  Add{,2,4,6} (4 alike) : Sum  Inputs=+-
  Add{1,3,5,7} (4 alike) : Sum  Inputs=-+
  Divide{,1..2,4..6,8..10,12..14} (12 alike) : Product  Inputs=**
  Divide{3,7,11,15} (4 alike) : Product  Inputs=***
  Trigonometric Function{,1,3..4,6..7,9..10} (8 alike) : Trigonometry  Operator=atan
  Trigonometric Function{2,5,8,11} (4 alike) : Trigonometry
  Fx01 : Outport  OutDataTypeStr=double  SampleTime=Ts
  Fx02 : Outport  Port=2  OutDataTypeStr=double  SampleTime=Ts
  Fx03 : Outport  Port=3  OutDataTypeStr=double  SampleTime=Ts
  Fx04 : Outport  Port=4  OutDataTypeStr=double  SampleTime=Ts
  wires:
  Divide13/1 -> Add7/1
  Trigonometric Function2/1 -> Divide3/3
  Divide11/1 -> Fx03/1  "Fx03"
  Divide7/1 -> Fx02/1  "Fx02"
  Divide1/1 -> Add1/1
  Trigonometric Function/1 -> Add/2
  Divide15/1 -> Fx04/1  "Fx04"
  Add/1 -> Divide1/2
  Divide/1 -> Add1/2, Add/1, Trigonometric Function/1
  k_f1/1 -> Divide/2
  k_r4/1 -> Divide12/2
  k_r3/1 -> Divide8/2
  Divide6/1 -> Trigonometric Function5/1
  Divide4/1 -> Add3/2, Add2/1, Trigonometric Function3/1
  Divide5/1 -> Add3/1
  Trigonometric Function3/1 -> Add2/2
  Add2/1 -> Divide5/2
  E_x_f/1 -> Divide5/1, Divide1/1
  B_x_f/1 -> Divide4/1, Divide/1
  Trigonometric Function4/1 -> Divide6/2
  C_x_f/1 -> Divide6/1, Divide2/1
  Trigonometric Function5/1 -> Divide7/3
  Add3/1 -> Trigonometric Function4/1
  C_x_r/1 -> Divide14/1, Divide10/1
  B_x_r/1 -> Divide12/1, Divide8/1
  E_x_r/1 -> Divide9/1, Divide13/1
  mu_x_r/1 -> Divide15/1, Divide11/1
  Fz2/1 -> Divide7/2
  mu_x_f/1 -> Divide7/1, Divide3/1
  k_f2/1 -> Divide4/2
  Fz1/1 -> Divide3/2
  Fz3/1 -> Divide11/2
  Add1/1 -> Trigonometric Function1/1
  Add4/1 -> Divide9/2
  Divide8/1 -> Add5/2, Add4/1, Trigonometric Function6/1
  Trigonometric Function8/1 -> Divide11/3
  Add5/1 -> Trigonometric Function7/1
  Trigonometric Function6/1 -> Add4/2
  Divide10/1 -> Trigonometric Function8/1
  Trigonometric Function7/1 -> Divide10/2
  Fz4/1 -> Divide15/2
  Divide9/1 -> Add5/1
  Trigonometric Function1/1 -> Divide2/2
  Divide3/1 -> Fx01/1  "Fx01"
  Divide2/1 -> Trigonometric Function2/1
  Trigonometric Function10/1 -> Divide14/2
  Trigonometric Function9/1 -> Add6/2
  Divide14/1 -> Trigonometric Function11/1
  Divide12/1 -> Add7/2, Add6/1, Trigonometric Function9/1
  Trigonometric Function11/1 -> Divide15/3
  Add7/1 -> Trigonometric Function10/1
  Add6/1 -> Divide13/2

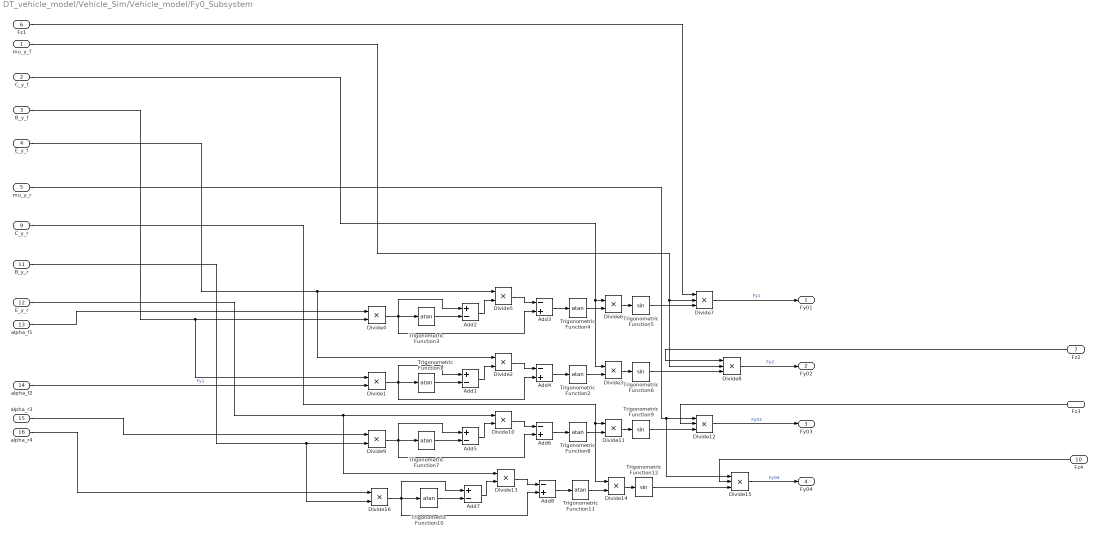
== system DT_vehicle_model/Vehicle_Sim/Vehicle_model/Fy0_Subsystem ==
  mu_y_f : Inport  OutDataTypeStr=double  SampleTime=Ts
  C_y_f : Inport  Port=2  OutDataTypeStr=double  SampleTime=Ts
  B_y_f : Inport  Port=3  OutDataTypeStr=double  SampleTime=Ts
  E_y_f : Inport  Port=4  OutDataTypeStr=double  SampleTime=Ts
  mu_y_r : Inport  Port=5  OutDataTypeStr=double  SampleTime=Ts
  Fz1 : Inport  Port=6  OutDataTypeStr=double  SampleTime=Ts
  Fz2 : Inport  Port=7  OutDataTypeStr=double  SampleTime=Ts
  Fz3 : Inport  Port=8  OutDataTypeStr=double  SampleTime=Ts
  C_y_r : Inport  Port=9  OutDataTypeStr=double  SampleTime=Ts
  Fz4 : Inport  Port=10  OutDataTypeStr=double  SampleTime=Ts
  B_y_r : Inport  Port=11  OutDataTypeStr=double  SampleTime=Ts
  E_y_r : Inport  Port=12  OutDataTypeStr=double  SampleTime=Ts
  alpha_f1 : Inport  Port=13  OutDataTypeStr=double  SampleTime=Ts
  alpha_f2 : Inport  Port=14  OutDataTypeStr=double  SampleTime=Ts
  alpha_r3 : Inport  Port=15  OutDataTypeStr=double  SampleTime=Ts
  alpha_r4 : Inport  Port=16  OutDataTypeStr=double  SampleTime=Ts
  Add{1..2,5,7} (4 alike) : Sum  Inputs=+-
  Add{3..4,6,8} (4 alike) : Sum  Inputs=-+
  Divide{1..6,9..11,13..14,16} (12 alike) : Product  Inputs=**
  Divide{7..8,12,15} (4 alike) : Product  Inputs=***
  Trigonometric Function{1..4,7..8,10..11} (8 alike) : Trigonometry  Operator=atan
  Trigonometric Function{5..6,9,12} (4 alike) : Trigonometry
  Fy01 : Outport  OutDataTypeStr=double  SampleTime=Ts
  Fy02 : Outport  Port=2  OutDataTypeStr=double  SampleTime=Ts
  Fy03 : Outport  Port=3  OutDataTypeStr=double  SampleTime=Ts
  Fy04 : Outport  Port=4  OutDataTypeStr=double  SampleTime=Ts
  wires:
  Add6/1 -> Trigonometric Function8/1
  Trigonometric Function9/1 -> Divide12/3
  alpha_r3/1 -> Divide9/1
  alpha_r4/1 -> Divide16/1
  C_y_f/1 -> Divide6/1, Divide3/1
  B_y_f/1 -> Divide4/2, Divide1/1
  alpha_f1/1 -> Divide4/1
  E_y_r/1 -> Divide13/1, Divide10/1
  B_y_r/1 -> Divide16/2, Divide9/2
  mu_y_r/1 -> Divide12/1, Divide15/1
  E_y_f/1 -> Divide5/1, Divide2/1
  mu_y_f/1 -> Divide8/2, Divide7/2
  Trigonometric Function1/1 -> Add1/2
  Add1/1 -> Divide2/2
  Trigonometric Function6/1 -> Divide8/3
  Trigonometric Function2/1 -> Divide3/2
  Divide1/1 -> Add4/2, Add1/1, Trigonometric Function1/1
  Divide3/1 -> Trigonometric Function6/1
  Divide2/1 -> Add4/1
  Add4/1 -> Trigonometric Function2/1
  Fz4/1 -> Divide15/2
  Fz3/1 -> Divide12/2
  Fz2/1 -> Divide8/1
  Fz1/1 -> Divide7/1
  C_y_r/1 -> Divide14/1, Divide11/1
  Divide15/1 -> Fy04/1  "Fy04"
  Trigonometric Function12/1 -> Divide15/3
  Add8/1 -> Trigonometric Function11/1
  Divide16/1 -> Add8/2, Add7/1, Trigonometric Function10/1
  Trigonometric Function11/1 -> Divide14/2
  Add7/1 -> Divide13/2
  Divide13/1 -> Add8/1
  Divide14/1 -> Trigonometric Function12/1
  Trigonometric Function10/1 -> Add7/2
  Divide12/1 -> Fy03/1  "Fy03"
  Divide9/1 -> Add6/2, Add5/1, Trigonometric Function7/1
  Trigonometric Function7/1 -> Add5/2
  Add5/1 -> Divide10/2
  Trigonometric Function5/1 -> Divide7/3
  Divide11/1 -> Trigonometric Function9/1
  Divide6/1 -> Trigonometric Function5/1
  Add3/1 -> Trigonometric Function4/1
  Trigonometric Function3/1 -> Add2/2
  Divide10/1 -> Add6/1
  Add2/1 -> Divide5/2
  Trigonometric Function4/1 -> Divide6/2
  Divide4/1 -> Add3/2, Add2/1, Trigonometric Function3/1
  Divide5/1 -> Add3/1
  Trigonometric Function8/1 -> Divide11/2
  Divide7/1 -> Fy01/1  "Fy1"
  Divide8/1 -> Fy02/1  "Fy2"
  alpha_f2/1 -> Divide1/2  "Fy1"

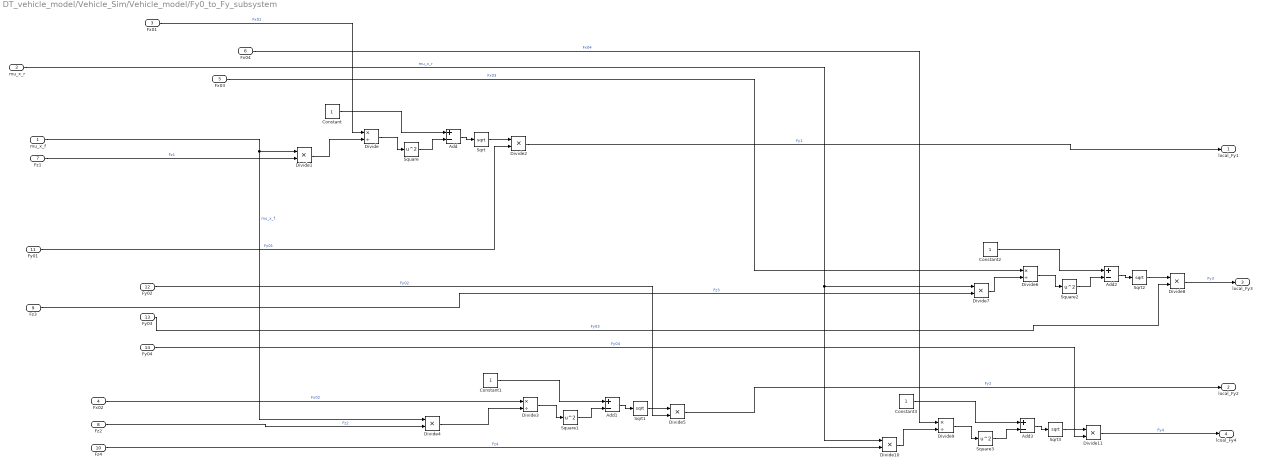
== system DT_vehicle_model/Vehicle_Sim/Vehicle_model/Fy0_to_Fy_subsystem ==
  mu_x_f : Inport  OutDataTypeStr=double  SampleTime=Ts
  mu_x_r : Inport  Port=2  OutDataTypeStr=double  SampleTime=Ts
  Fx01 : Inport  Port=3  OutDataTypeStr=double  SampleTime=Ts
  Fx02 : Inport  Port=4  OutDataTypeStr=double  SampleTime=Ts
  Fx03 : Inport  Port=5  OutDataTypeStr=double  SampleTime=Ts
  Fx04 : Inport  Port=6  OutDataTypeStr=double  SampleTime=Ts
  Fz1 : Inport  Port=7  OutDataTypeStr=double  SampleTime=Ts
  Fz2 : Inport  Port=8  OutDataTypeStr=double  SampleTime=Ts
  Fz3 : Inport  Port=9  OutDataTypeStr=double  SampleTime=Ts
  Fz4 : Inport  Port=10  OutDataTypeStr=double  SampleTime=Ts
  Fy01 : Inport  Port=11  OutDataTypeStr=double  SampleTime=Ts
  Fy02 : Inport  Port=12  OutDataTypeStr=double  SampleTime=Ts
  Fy03 : Inport  Port=13  OutDataTypeStr=double  SampleTime=Ts
  Fy04 : Inport  Port=14  OutDataTypeStr=double  SampleTime=Ts
  Add{,1..3} (4 alike) : Sum  Inputs=+-
  Constant{,1..3} (4 alike) : Constant
  Divide{,3,6,9} (4 alike) : Product  Inputs=*/
  Divide{1..2,4..5,7..8,10..11} (8 alike) : Product  Inputs=**
  Sqrt{,1..3} (4 alike) : Sqrt  SaturateOnIntegerOverflow=on
  Square{,1..3} (4 alike) : Math  Operator=square  RndMeth=Zero  SaturateOnIntegerOverflow=on
  local_Fy1 : Outport  OutDataTypeStr=double  SampleTime=Ts
  local_Fy2 : Outport  Port=2  OutDataTypeStr=double  SampleTime=Ts
  local_Fy3 : Outport  Port=3  OutDataTypeStr=double  SampleTime=Ts
  lcoal_Fy4 : Outport  Port=4  OutDataTypeStr=double  SampleTime=Ts
  wires:
  Divide1/1 -> Divide/2
  Divide/1 -> Square/1
  Constant/1 -> Add/1
  Divide2/1 -> local_Fy1/1  "Fy1"
  Divide11/1 -> lcoal_Fy4/1  "Fy4"
  Fz4/1 -> Divide10/2  "Fz4"
  mu_x_f/1 -> Divide4/1, Divide1/1  "mu_x_f"
  Fx04/1 -> Divide9/1  "Fx04"
  Fx01/1 -> Divide/1  "Fx01"
  Fz3/1 -> Divide7/2  "Fz3"
  Fx02/1 -> Divide3/1  "Fx02"
  mu_x_r/1 -> Divide10/1, Divide7/1  "mu_x_r"
  Fx03/1 -> Divide6/1  "Fx03"
  Fz1/1 -> Divide1/2  "Fz1"
  Fz2/1 -> Divide4/2  "Fz2"
  Square2/1 -> Add2/2
  Divide6/1 -> Square2/1
  Sqrt2/1 -> Divide8/1
  Constant2/1 -> Add2/1
  Sqrt3/1 -> Divide11/1
  Constant3/1 -> Add3/1
  Add3/1 -> Sqrt3/1
  Divide9/1 -> Square3/1
  Square3/1 -> Add3/2
  Add/1 -> Sqrt/1
  Square/1 -> Add/2
  Divide10/1 -> Divide9/2
  Divide8/1 -> local_Fy3/1  "Fy3"
  Sqrt/1 -> Divide2/1
  Divide4/1 -> Divide3/2
  Square1/1 -> Add1/2
  Divide3/1 -> Square1/1
  Constant1/1 -> Add1/1
  Fy02/1 -> Divide5/2  "Fy02"
  Add1/1 -> Sqrt1/1
  Sqrt1/1 -> Divide5/1
  Divide7/1 -> Divide6/2
  Add2/1 -> Sqrt2/1
  Fy03/1 -> Divide8/2  "Fy03"
  Divide5/1 -> local_Fy2/1  "Fy2"
  Fy01/1 -> Divide2/2  "Fy01"
  Fy04/1 -> Divide11/2  "Fy04"

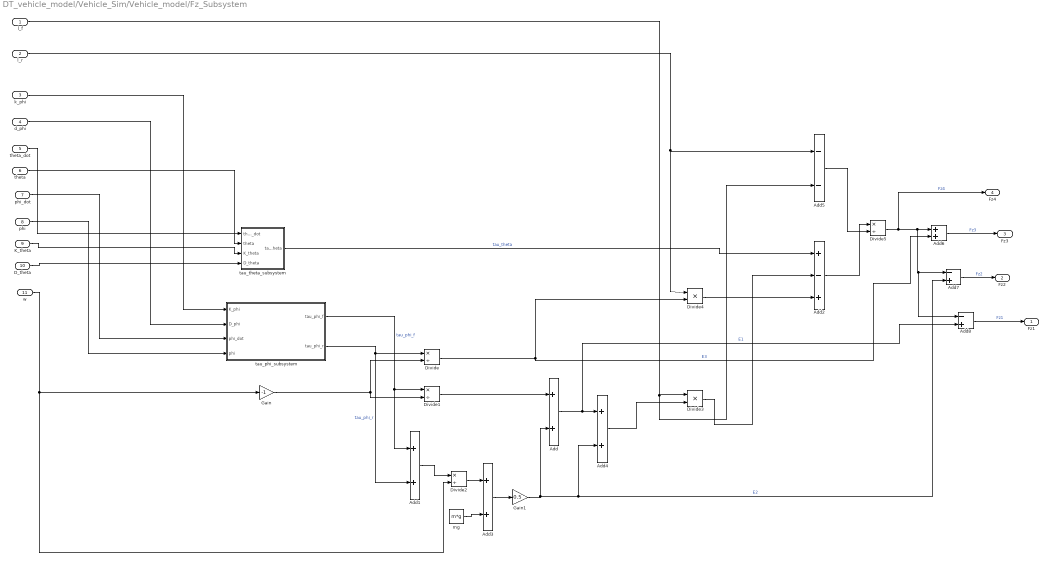
== system DT_vehicle_model/Vehicle_Sim/Vehicle_model/Fz_Subsystem ==
  l_f : Inport  OutDataTypeStr=double  SampleTime=Ts
  l_r : Inport  Port=2  OutDataTypeStr=double  SampleTime=Ts
  k_phi : Inport  Port=3  OutDataTypeStr=double  SampleTime=Ts
  d_phi : Inport  Port=4  OutDataTypeStr=double  SampleTime=Ts
  theta_dot : Inport  Port=5  OutDataTypeStr=double  SampleTime=Ts
  theta : Inport  Port=6  OutDataTypeStr=double  SampleTime=Ts
  phi_dot : Inport  Port=7  OutDataTypeStr=double  SampleTime=Ts
  phi : Inport  Port=8  OutDataTypeStr=double  SampleTime=Ts
  K_theta : Inport  Port=9  OutDataTypeStr=double  SampleTime=Ts
  D_theta : Inport  Port=10  OutDataTypeStr=double  SampleTime=Ts
  w : Inport  Port=11  OutDataTypeStr=double  SampleTime=Ts
  Add{,1,3..4,6} (5 alike) : Sum
  Add2 : Sum  Inputs=+-+
  Add5 : Sum  Inputs=--
  Add7 : Sum  Inputs=-+
  Add8 : Sum  Inputs=-+
  Divide{,1..2,5} (4 alike) : Product  Inputs=*/
  Divide3 : Product  Inputs=**
  Divide4 : Product  Inputs=**
  Gain : Gain  Gain=-1  OutDataTypeStr=double
  Gain1 : Gain  Gain=0.5
  mg : Constant  Value=m*g
  tau_phi_subsystem : Subsystem
  tau_theta_subsystem : Subsystem
  Fz1 : Outport  OutDataTypeStr=double  SampleTime=Ts
  Fz2 : Outport  Port=2  OutDataTypeStr=double  SampleTime=Ts
  Fz3 : Outport  Port=3  OutDataTypeStr=double  SampleTime=Ts
  Fz4 : Outport  Port=4  OutDataTypeStr=double  SampleTime=Ts
  wires:
  phi/1 -> tau_phi_subsystem/4(phi)
  theta/1 -> tau_theta_subsystem/2(theta)
  phi_dot/1 -> tau_phi_subsystem/3(phi_dot)
  w/1 -> Divide2/2, Gain/1
  Add1/1 -> Divide2/1
  Divide2/1 -> Add3/1
  Add2/1 -> Divide5/1
  d_phi/1 -> tau_phi_subsystem/2(D_phi)
  D_theta/1 -> tau_theta_subsystem/4(D_theta)
  l_r/1 -> Divide4/1, Add5/1
  theta_dot/1 -> tau_theta_subsystem/1(theta_dot)
  tau_theta_subsystem/1(tau_theta) -> Add2/1  "tau_theta"
  K_theta/1 -> tau_theta_subsystem/3(K_theta)
  Add8/1 -> Fz1/1  "Fz1"
  Add/1 -> Add8/2, Add4/1  "E1"
  Divide3/1 -> Add2/2
  Divide5/1 -> Fz4/1, Add8/1, Add7/1, Add6/1  "Fz4"
  Add3/1 -> Gain1/1
  Add5/1 -> Divide5/2
  Gain1/1 -> Add7/2, Add4/2, Add/2  "E2"
  Add4/1 -> Divide3/2
  Add6/1 -> Fz3/1  "Fz3"
  Divide/1 -> Divide4/2, Add6/2  "E3"
  mg/1 -> Add3/2
  Divide4/1 -> Add2/3
  Divide1/1 -> Add/1
  k_phi/1 -> tau_phi_subsystem/1(K_phi)
  l_f/1 -> Add5/2, Divide3/1
  Add7/1 -> Fz2/1  "Fz2"
  tau_phi_subsystem/1(tau_phi_f) -> Divide1/1, Add1/1  "tau_phi_f"
  tau_phi_subsystem/2(tau_phi_r) -> Add1/2, Divide/1  "tau_phi_r"
  Gain/1 -> Divide1/2, Divide/2

== system DT_vehicle_model/Vehicle_Sim/Vehicle_model/Pacjeka_parameters_Subsystem ==
  surface_condition : Inport  OutDataTypeStr=double  SampleTime=Ts
  Ashphalt_condition_subsystem : Subsystem  TreatAsAtomicUnit=on
  Demux : Demux  Outputs=2
  If : If  IfExpression=(u1==1)
  Merge : Merge
  Snow_condition_subsystem : Subsystem  TreatAsAtomicUnit=on
  front : Outport  OutDataTypeStr=double  SampleTime=Ts
  rear : Outport  Port=2  OutDataTypeStr=double  SampleTime=Ts
  wires:
  Demux/2 -> rear/1  "rear"
  Merge/1 -> Demux/1
  If/1 -> Ashphalt_condition_subsystem/Action
  If/2 -> Snow_condition_subsystem/Action
  Demux/1 -> front/1  "front"
  surface_condition/1 -> If/1
  Ashphalt_condition_subsystem/1(Out1) -> Merge/1
  Snow_condition_subsystem/1(Out1) -> Merge/2

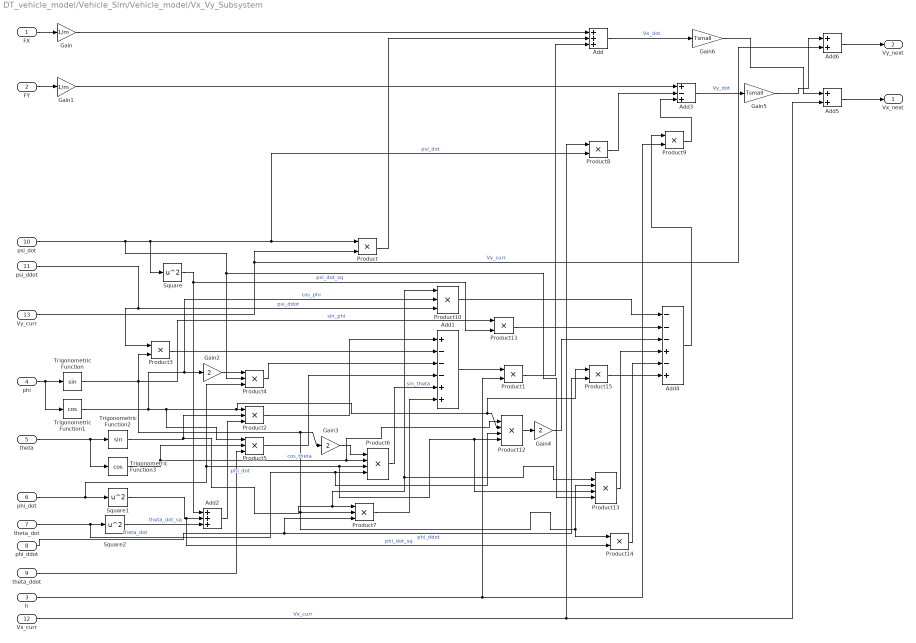
== system DT_vehicle_model/Vehicle_Sim/Vehicle_model/Vx_Vy_Subsystem ==
  FX : Inport  OutDataTypeStr=double  SampleTime=Ts
  FY : Inport  Port=2  OutDataTypeStr=double  SampleTime=Ts
  h : Inport  Port=3  OutDataTypeStr=double  SampleTime=Ts
  phi : Inport  Port=4  OutDataTypeStr=double  SampleTime=Ts
  theta : Inport  Port=5  OutDataTypeStr=double  SampleTime=Ts
  phi_dot : Inport  Port=6  OutDataTypeStr=double  SampleTime=Ts
  theta_dot : Inport  Port=7  OutDataTypeStr=double  SampleTime=Ts
  phi_ddot : Inport  Port=8  OutDataTypeStr=double  SampleTime=Ts
  theta_ddot : Inport  Port=9  OutDataTypeStr=double  SampleTime=Ts
  psi_dot : Inport  Port=10  OutDataTypeStr=double  SampleTime=Ts
  psi_ddot : Inport  Port=11  OutDataTypeStr=double  SampleTime=Ts
  Vx_curr : Inport  Port=12  OutDataTypeStr=double  SampleTime=Tsmall
  Vy_curr : Inport  Port=13  OutDataTypeStr=double  SampleTime=Tsmall
  Add : Sum  Inputs=+++
  Add1 : Sum  Inputs=+---++
  Add2 : Sum  Inputs=+++
  Add3 : Sum  Inputs=+-+
  Add4 : Sum  Inputs=---+-+
  Add5 : Sum
  Add6 : Sum
  Gain : Gain  Gain=1/m
  Gain1 : Gain  Gain=1/m
  Gain2 : Gain  Gain=2
  Gain3 : Gain  Gain=2
  Gain4 : Gain  Gain=2
  Gain5 : Gain  Gain=Tsmall
  Gain6 : Gain  Gain=Tsmall
  Product{,1,3,8..9,11,14..15} (8 alike) : Product
  Product{2,4..5,7,10} (5 alike) : Product  Inputs=3
  Product12 : Product  Inputs=4
  Product13 : Product  Inputs=4
  Product6 : Product  Inputs=4
  Square : Math  Operator=square  RndMeth=Zero  SaturateOnIntegerOverflow=on
  Square1 : Math  Operator=square  RndMeth=Zero  SaturateOnIntegerOverflow=on
  Square2 : Math  Operator=square  RndMeth=Zero  SaturateOnIntegerOverflow=on
  Trigonometric Function : Trigonometry
  Trigonometric Function1 : Trigonometry  Operator=cos
  Trigonometric Function2 : Trigonometry
  Trigonometric Function3 : Trigonometry  Operator=cos
  Vx_next : Outport  OutDataTypeStr=double  SampleTime=Tsmall
  Vy_next : Outport  Port=2  OutDataTypeStr=double  SampleTime=Tsmall
  wires:
  FX/1 -> Gain/1
  FY/1 -> Gain1/1
  Gain/1 -> Add/1
  psi_dot/1 -> Product4/2, Product13/4, Square/1, Product8/2, Product/1  "psi_dot"
  Product/1 -> Add/2
  Vy_curr/1 -> Add6/2, Product/2  "Vy_curr"
  Product1/1 -> Add/3
  phi/1 -> Trigonometric Function1/1, Trigonometric Function/1
  theta/1 -> Trigonometric Function3/1, Trigonometric Function2/1
  Add1/1 -> Product1/1
  h/1 -> Product9/2, Product1/2
  Add2/1 -> Product2/3
  Square/1 -> Product11/2, Add2/1  "psi_dot_sq"
  Square1/1 -> Product14/2, Add2/2  "phi_dot_sq"
  phi_dot/1 -> Product13/3, Product12/4, Product6/3, Product4/3, Square1/1  "phi_dot"
  Square2/1 -> Add2/3  "theta_dot_sq"
  theta_dot/1 -> Product12/3, Product6/4, Square2/1  "theta_dot"
  Product2/1 -> Add1/1
  Trigonometric Function/1 -> Product11/1, Product14/1, Product13/2, Product7/2, Gain3/1, Product3/2  "sin_phi"
  psi_ddot/1 -> Product10/3, Product3/1  "psi_ddot"
  Product3/1 -> Add1/2
  Gain2/1 -> Product4/1
  Product4/1 -> Add1/3
  Trigonometric Function3/1 -> Product5/2, Product12/1, Product6/2  "cos_theta"
  theta_ddot/1 -> Product5/3
  Product5/1 -> Add1/4
  Product6/1 -> Add1/5
  Gain3/1 -> Product6/1
  phi_ddot/1 -> Product15/2, Product7/3  "phi_ddot"
  Product7/1 -> Add1/6
  Add/1 -> Gain6/1  "Vx_dot"
  Gain1/1 -> Add3/1
  Vx_curr/1 -> Add5/2, Product8/1  "Vx_curr"
  Product8/1 -> Add3/2
  Add4/1 -> Product9/1
  Product9/1 -> Add3/3
  Product10/1 -> Add4/1
  Trigonometric Function2/1 -> Product13/1, Product10/1, Product7/1, Product2/2  "sin_theta"
  Trigonometric Function1/1 -> Product10/2, Gain2/1, Product5/1, Product15/1, Product12/2, Product2/1  "cos_phi"
  Product11/1 -> Add4/2
  Product12/1 -> Gain4/1
  Gain4/1 -> Add4/3
  Product13/1 -> Add4/4
  Product14/1 -> Add4/5
  Product15/1 -> Add4/6
  Add3/1 -> Gain5/1  "Vy_dot"
  Gain5/1 -> Add6/1
  Add5/1 -> Vx_next/1
  Gain6/1 -> Add5/1
  Add6/1 -> Vy_next/1
